simulink model "sampling_bandpass"  (R2020b)
settings: Solver=ode45  StartTime=0.0  StopTime=11  RelTol=1e-3  EnableMultiTasking=on
libraries: dsparch4 x3
settings Model: Creator=morelos_zaragoza  LastModifiedBy=14083
settings DataIOCC: LimitDataPoints=on  SaveFormat=Array  SignalLoggingSaveFormat=ModelDataLogs  ReturnWorkspaceOutputs=off
settings OptimizationCC: ExpressionDepthLimit=2147483647  InitFltsAndDblsToZero=on  LifeSpan=inf
settings DebuggingCC: SaveWithParameterizedLinksMsg=none  UnderspecifiedInitializationDetection=Classic  MergeDetectMultiDrivingBlocksExec=none  SignalResolutionControl=TryResolveAllWithWarning  SolverPrmCheckMsg=warning  MultiTaskDSMMsg=warning  MultiTaskCondExecSysMsg=none  FcnCallInpInsideContextMsg=warning  StateNameClashWarn=warning  SFUnexpectedBacktrackingDiag=warning  SFNoUnconditionalDefaultTransitionDiag=warning  SFExecutionAtInitializationDiag=none  ArithmeticOperatorsInVariantConditions=warning
settings HardwareCC: ProdBitPerPointer=32  ProdBitPerSizeT=32  ProdBitPerPtrDiffT=32  ProdLargestAtomicFloat=None  ProdIntDivRoundTo=Undefined  ProdEndianess=Unspecified  ProdWordSize=32  ProdHWDeviceType=32-bit Generic
settings ModelReferenceCC: PropagateSignalLabelsOutOfModel=off
settings SFSimCC: SimUseLocalCustomCode=off  CustomCodeUndefinedFunction=UseInterfaceOnly
settings RTWCC: RTWUseLocalCustomCode=off
settings CodeAppCC: StateflowObjectComments=on
settings GRTTargetCC: TargetFcnLib=ansi_tfl_tmw.mat  TargetLangStandard=C89/C90 (ANSI)  CombineOutputUpdateFcns=off  GRTInterface=on
settings ConfigComp: CovMetricSettings=dw  CovSaveCumulativeToWorkspaceVar=on  CovSaveSingleToWorkspaceVar=on  CovExternalEMLEnable=off

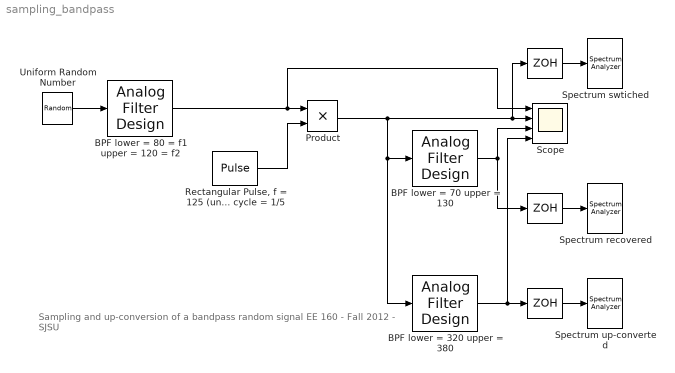
== system sampling_bandpass ==
  note: Sampling and up-conversion of a bandpass random signal
      | EE 160 - Fall 2012 - SJSU
  " " : ZeroOrderHold  SampleTime=1/2000
  "  " : ZeroOrderHold  SampleTime=1/2000
  "     " : ZeroOrderHold  SampleTime=1/2000
  BPF lower = 320 upper = 380 : dsparch4/Analog Filter Design  method=Chebyshev II  filttype=Bandpass  N=12  Wlo=2*pi*320  Whi=2*pi*380  Rp=2  Rs=40
  BPF lower = 70 upper = 130 : dsparch4/Analog Filter Design  method=Chebyshev II  filttype=Bandpass  N=12  Wlo=2*pi*70  Whi=2*pi*130  Rp=2  Rs=40
  BPF lower = 80 = f1 upper = 120 = f2 : dsparch4/Analog Filter Design  method=Chebyshev II  filttype=Bandpass  N=12  Wlo=2*pi*80  Whi=2*pi*120  Rp=2  Rs=40
  Product : Product  RndMeth=Zero
  "Rectangular Pulse, f = 125 (undersampling factor k = 2) Dute cycle = 1/5" : DiscretePulseGenerator  PulseType=Time based  Period=1/125  PulseWidth=20  SampleTime=1e-2/2)
  Scope : Scope  NumInputPorts=4
  Spectrum recovered : SpectrumAnalyzer
  Spectrum swtiched : SpectrumAnalyzer
  Spectrum up-converted : SpectrumAnalyzer
  Uniform Random Number : UniformRandomNumber  Seed=23453  SampleTime=1/240
  wires:
  "Rectangular Pulse, f = 125 (undersampling factor k = 2) Dute cycle = 1/5"/1 -> Product/2
  Product/1 -> "  "/1, Scope/2, BPF lower = 70 upper = 130/1, BPF lower = 320 upper = 380/1
  "  "/1 -> Spectrum swtiched/1
  BPF lower = 80 = f1 upper = 120 = f2/1 -> Product/1, Scope/1
  BPF lower = 70 upper = 130/1 -> Scope/3, " "/1
  " "/1 -> Spectrum recovered/1
  Uniform Random Number/1 -> BPF lower = 80 = f1 upper = 120 = f2/1
  "     "/1 -> Spectrum up-converted/1
  BPF lower = 320 upper = 380/1 -> "     "/1, Scope/4
